simulink model "Buck_Control_Sim"  (R2023b)
settings: Solver=ode23t  StartTime=0.0  StopTime=20e-3  RelTol=1e-6
undefined symbols (not defined in the file): C, C1_dl_Den, C1_dl_Num, C1_sl_Den, C1_sl_Num, C2_dl_Den, C2_dl_Num, C2_dlh_Den, C2_dlh_Num, fs, L, R, Vg
libraries: spsSeriesRLCBranchLib x9, spsCurrentMeasurementLib x3, spsDiodeLib x3, spsIdealSwitchLib x3, spsMeanLib x3, eePwmGenerator x3, spsDCVoltageSourceLib x3, spsVoltageMeasurementLib x3, slpidlib x1, sps_lib x1
settings Model: Creator=Lucas  LastModifiedBy=Lucas
settings SolverCC: ZeroCrossAlgorithm=Adaptive
settings DebuggingCC: IgnoredZcDiagnostic=none

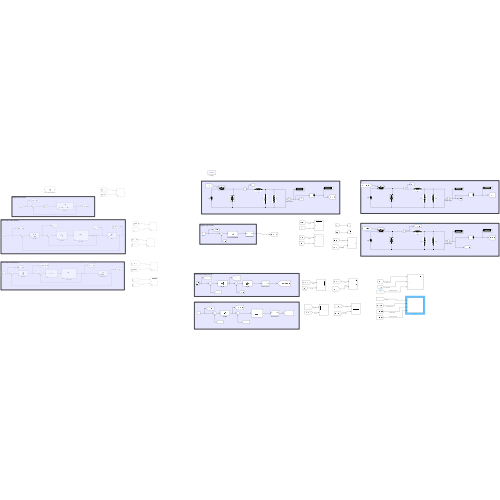
[thumbnail: Simulink's stored preview of the top-level diagram]
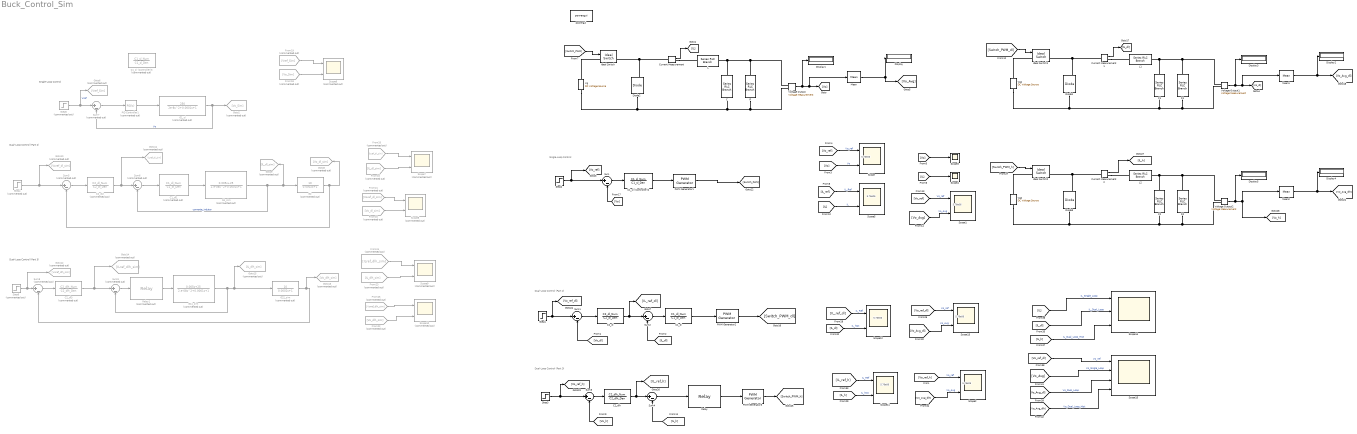
== system Buck_Control_Sim ==
  note: 5.76e06
  note: Single-Loop Control
  note: Dual-Loop Control (Part 2)
  note: 5.76e06
  note: Dual-Loop Control (Part 3)
  note: 5.76e06
  note: Dual-Loop Control (Part 2)
  note: Single-Loop Control
  note: Dual-Loop Control (Part 3)
  note: 5.76e06
  note: 5.76e06
  note: 5.76e06
  note: 5.76e06
  C : spsSeriesRLCBranchLib/Series RLC Branch  LConnTagsString=__new0  RConnTagsString=__new0  BranchType=C  Resistance=1  Inductance=L  SetiL0=off  InitialCurrent=0  Capacitance=C  Setx0=off  InitialVoltage=0  Measurements=None
  C1 : spsSeriesRLCBranchLib/Series RLC Branch  LConnTagsString=__new0  RConnTagsString=__new0  BranchType=C  Resistance=1  Inductance=L  SetiL0=off  InitialCurrent=0  Capacitance=C  Setx0=off  InitialVoltage=0  Measurements=None
  C1_dl : TransferFcn  Numerator=C1_dl_Num  Denominator=C1_dl_Den
  C1_dl1 : TransferFcn  Commented=on  Numerator=C1_dl_Num  Denominator=C1_dl_Den
  C1_sl (Controller)2 : TransferFcn  Numerator=C1_sl_Num  Denominator=C1_sl_Den
  C1_sl (Controller)3 : TransferFcn  Commented=on  Numerator=C1_sl_Num  Denominator=C1_sl_Den
  C2 : spsSeriesRLCBranchLib/Series RLC Branch  LConnTagsString=__new0  RConnTagsString=__new0  BranchType=C  Resistance=1  Inductance=L  SetiL0=off  InitialCurrent=0  Capacitance=C  Setx0=off  InitialVoltage=0  Measurements=None
  C2_dl : TransferFcn  Numerator=C2_dl_Num  Denominator=C2_dl_Den
  C2_dl2 : TransferFcn  Commented=on  Numerator=C2_dl_Num  Denominator=C2_dl_Den
  C2_dl3 : TransferFcn  Commented=on  Numerator=C2_dlh_Num  Denominator=C2_dlh_Den
  C2_dlh : TransferFcn  Numerator=C2_dlh_Num  Denominator=C2_dlh_Den
  Current Measurement : spsCurrentMeasurementLib/Current Measurement  PhasorSimulation=off  OutputType=Complex  PSBequivalent=0
  Current Measurement1 : spsCurrentMeasurementLib/Current Measurement  PhasorSimulation=off  OutputType=Complex  PSBequivalent=0
  Current Measurement2 : spsCurrentMeasurementLib/Current Measurement  PhasorSimulation=off  OutputType=Complex  PSBequivalent=0
  Diode1 : spsDiodeLib/Diode  Ron=0.00001  Lon=0  Vf=0  IC=0  UseSnubber=0  Rs=inf  Cs=inf  Measurements=on
  Diode2 : spsDiodeLib/Diode  Ron=0.00001  Lon=0  Vf=0  IC=0  UseSnubber=0  Rs=inf  Cs=inf  Measurements=on
  Diode3 : spsDiodeLib/Diode  Ron=0.00001  Lon=0  Vf=0  IC=0  UseSnubber=0  Rs=inf  Cs=inf  Measurements=on
  Display{,1..5} (6 alike) : Display
  From15 : From  Commented=on  GotoTag=Vo_dl_sim
  From16 : From  Commented=on  GotoTag=IL_dl_sim
  From18 : From  Commented=on  GotoTag=Vo_Sim
  From19 : From  Commented=on  GotoTag=Vref_Sim
  From20 : From  Commented=on  GotoTag=ILref_dl_sim
  From21 : From  Commented=on  GotoTag=Voref_dl_sim
  From22 : From  Commented=on  GotoTag=Vo_dlh_sim
  From23 : From  Commented=on  GotoTag=IL_dlh_sim
  From24 : From  Commented=on  GotoTag=ILref_dlh_sim
  From25 : From  Commented=on  GotoTag=Voref_dlh_sim
  G11_sim : TransferFcn  Commented=on  Numerator=[0 0.005 25]  Denominator=[2.e-08 0.0001 1]
  G1_sim : TransferFcn  Commented=on  Numerator=[0 0.005 25]  Denominator=[2.e-08 0.0001 1]
  G1_sl : TransferFcn  Commented=on  Numerator=[250]  Denominator=[2e-8 0.0001 1]
  G2 : TransferFcn  Commented=on  Numerator=[0,10]  Denominator=[0.0002 1]
  G22_sim : TransferFcn  Commented=on  Numerator=[0,10]  Denominator=[0.0002 1]
  Goto10 : Goto  Commented=on  GotoTag=Voref_dl_sim
  Goto11 : Goto  Commented=on  GotoTag=ILref_dl_sim
  Goto12 : Goto  Commented=on  GotoTag=Voref_dlh_sim
  Goto13 : Goto  Commented=on  GotoTag=Vo_dlh_sim
  Goto14 : Goto  Commented=on  GotoTag=ILref_dlh_sim
  Goto15 : Goto  Commented=on  GotoTag=IL_dlh_sim
  Goto2 : Goto  Commented=on  GotoTag=Vo_Sim
  Goto6 : Goto  Commented=on  GotoTag=Vref_Sim
  Goto8 : Goto  Commented=on  GotoTag=Vo_dl_sim
  Goto9 : Goto  Commented=on  GotoTag=IL_dl_sim
  Ideal Switch : spsIdealSwitchLib/Ideal Switch  Ron=0.001  Lon=0  IC=0  Rs=1e5  Cs=inf  Measurements=on
  Ideal Switch1 : spsIdealSwitchLib/Ideal Switch  Ron=0.001  Lon=0  IC=0  Rs=1e5  Cs=inf  Measurements=on
  Ideal Switch2 : spsIdealSwitchLib/Ideal Switch  Ron=0.001  Lon=0  IC=0  Rs=1e5  Cs=inf  Measurements=on
  L : spsSeriesRLCBranchLib/Series RLC Branch  LConnTagsString=__new0  RConnTagsString=__new0  BranchType=L  Resistance=1  Inductance=L  SetiL0=off  InitialCurrent=0  Capacitance=1e-6  Setx0=off  InitialVoltage=0  Measurements=None
  L1 : spsSeriesRLCBranchLib/Series RLC Branch  LConnTagsString=__new0  RConnTagsString=__new0  BranchType=L  Resistance=1  Inductance=L  SetiL0=off  InitialCurrent=0  Capacitance=1e-6  Setx0=off  InitialVoltage=0  Measurements=None
  L2 : spsSeriesRLCBranchLib/Series RLC Branch  LConnTagsString=__new0  RConnTagsString=__new0  BranchType=L  Resistance=1  Inductance=L  SetiL0=off  InitialCurrent=0  Capacitance=1e-6  Setx0=off  InitialVoltage=0  Measurements=None
  Mean : spsMeanLib/Mean  Freq=fs  Vinit=0  Ts=0
  Mean1 : spsMeanLib/Mean  Freq=fs  Vinit=0  Ts=0
  Mean2 : spsMeanLib/Mean  Freq=fs  Vinit=0  Ts=0
  PID Controller1 : slpidlib/PID Controller  Commented=on  Controller=PID  Form=Parallel  TimeDomain=Continuous-time  UseExternalTs=off  SampleTime=-1  IntegratorMethod=Forward Euler  FilterMethod=Forward Euler  ControllerParametersSource=internal  P=0  I=6.07  UseKiTs=off  D=0  N=100  UseFilter=on  TunerSelectOption=Transfer Function Based (PID Tuner App)  InitialConditionSource=internal  InitialConditionForIntegrator=0  InitialConditionForFilter=0  DifferentiatorICPrevScaledInput=0  ExternalReset=none  TrackingMode=off  Kt=1  LimitOutput=off  SatLimitsSource=internal  UpperSaturationLimit=inf  LowerSaturationLimit=-inf  LinearizeAsGain=on  AntiWindupMode=none  Kb=1  LimitIntegrator=off  UpperIntegratorSaturationLimit=inf  LowerIntegratorSaturationLimit=-inf  POutMin=[]  POutMax=[]  IOutMin=[]  IOutMax=[]  DOutMin=[]  DOutMax=[]  NOutMin=[]  NOutMax=[]  SumOutMin=[]  SumOutMax=[]  SaturationOutMin=[]  SaturationOutMax=[]  PParamMin=[]  PParamMax=[]  IParamMin=[]  IParamMax=[]  DParamMin=[]  DParamMax=[]  NParamMin=[]  NParamMax=[]  KbParamMin=[]  KbParamMax=[]  KtParamMin=[]  KtParamMax=[]  KbOutMin=[]  KbOutMax=[]  KtOutMin=[]  KtOutMax=[]  IntegratorOutMin=[]  IntegratorOutMax=[]  FilterOutMin=[]  FilterOutMax=[]  SumI1OutMin=[]  SumI1OutMax=[]  SumI2OutMin=[]  SumI2OutMax=[]  SumI3OutMin=[]  SumI3OutMax=[]  SumI4OutMin=[]  SumI4OutMax=[]  SumDOutMin=[]  SumDOutMax=[]  DifferentiatorOutMin=[]  DifferentiatorOutMax=[]  FilterDiffOutCoefMin=[]  FilterDiffOutCoefMax=[]  ReciprocalOutMin=[]  ReciprocalOutMax=[]  SumDenOutMin=[]  SumDenOutMax=[]  SumNumOutMin=[]  SumNumOutMax=[]  DivideOutMin=[]  DivideOutMax=[]  UdiffTsProdOutMin=[]  UdiffTsProdOutMax=[]  NTsProdOutMin=[]  NTsProdOutMax=[]  UintegralTsProdOutMin=[]  UintegralTsProdOutMax=[]  UngainTsProdOutMin=[]  UngainTsProdOutMax=[]  ClampingZeroOutDataTypeStr=Inherit: Inherit via back propagation  ClampingZeroOutMin=[]  ClampingZeroOutMax=[]  FilterDenConstantOutDataTypeStr=Inherit: Inherit via back propagation  FilterDenConstantOutMin=[]  FilterDenConstantOutMax=[]  PCopyOutDataTypeStr=Inherit: Inherit via back propagation  PCopyOutMin=[]  PCopyOutMax=[]  NCopyOutDataTypeStr=Inherit: Inherit via back propagation  NCopyOutMin=[]  NCopyOutMax=[]  IntegratorContinuousStateAttributes=''  IntegratorStateMustResolveToSignalObject=off  IntegratorRTWStateStorageClass=Auto  FilterContinuousStateAttributes=''  FilterStateMustResolveToSignalObject=off  FilterRTWStateStorageClass=Auto  ParallelPVariant=InternalParameters  IdealPVariant=Disabled  IVariant=InternalParameters  DVariant=InternalParameters  IntegratorVariant=Continuous  SatVariant=Disabled  AWVariant=Passthrough  PCopyVariant=Disabled  TRVariant=Disabled  FdbkBlocksVariant=Forward  IdealPFdbkVariant=Disabled  SatFdbkVariant=Disabled  DerivativeFilterVariant=ContFilter  NVariant=InternalParameters  NCopyVariant=Disabled  FilterICVariant=InternalICsFilter  IntegratorICVariant=InternalICs  ExternalResetVariant=Disabled  TRSumVariant=Passthrough  SumFdbkVariant=Disabled  SumVariant=Sum_PID  TsampFilterVariant=InternalTs  TsampNgainVariant=Passthrough  TsampIntegralVariant=Disabled_SignalSpec  ExternalSaturationOutDataTypeStr=Inherit: Same as second input
  PWM Generator1 : eePwmGenerator/PWM Generator  CarrCount=Up  Tper=1/fs  Tdelay=0  Ts=0
  PWM Generator2 : eePwmGenerator/PWM Generator  CarrCount=Up  Tper=1/fs  Tdelay=0  Ts=0
  PWM Generator3 : eePwmGenerator/PWM Generator  CarrCount=Up  Tper=1/fs  Tdelay=0  Ts=0
  R : spsSeriesRLCBranchLib/Series RLC Branch  LConnTagsString=__new0  RConnTagsString=__new0  BranchType=R  Resistance=R  Inductance=L  SetiL0=off  InitialCurrent=0  Capacitance=1e-6  Setx0=off  InitialVoltage=0  Measurements=None
  R1 : spsSeriesRLCBranchLib/Series RLC Branch  LConnTagsString=__new0  RConnTagsString=__new0  BranchType=R  Resistance=R  Inductance=L  SetiL0=off  InitialCurrent=0  Capacitance=1e-6  Setx0=off  InitialVoltage=0  Measurements=None
  R2 : spsSeriesRLCBranchLib/Series RLC Branch  LConnTagsString=__new0  RConnTagsString=__new0  BranchType=R  Resistance=R  Inductance=L  SetiL0=off  InitialCurrent=0  Capacitance=1e-6  Setx0=off  InitialVoltage=0  Measurements=None
  Relay : Relay  OnSwitchValue=0.1  OffSwitchValue=0  OnOutputValue=200
  Relay1 : Relay  Commented=on  OnSwitchValue=0.1  OffSwitchValue=0  OnOutputValue=200
  Scope{,1..2,5,11..13} (7 alike) : Scope  NumInputPorts=2
  Scope{6..10} (5 alike) : Scope  Commented=on  NumInputPorts=2
  Scope14 : Scope  NumInputPorts=3
  Scope15 : Scope  NumInputPorts=4
  Scope3 : Scope
  Scope4 : Scope
  Step1 : Step  Time=10e-3  Before=60  After=66  SampleTime=0
  Step2 : Step  Time=10e-3  Before=60  After=66  SampleTime=0
  Step3 : Step  Time=10e-3  Before=60  After=66  SampleTime=0
  Step4 : Step  Commented=on  Time=6e-3  Before=60  After=66  SampleTime=0
  Step5 : Step  Commented=on  Time=6e-3  Before=60  After=66  SampleTime=0
  Step6 : Step  Commented=on  Time=6e-3  Before=60  After=66  SampleTime=0
  Sum{,1..4} (5 alike) : Sum  Inputs=|+-
  Sum{5..9} (5 alike) : Sum  Commented=on  Inputs=|+-
  Vg : spsDCVoltageSourceLib/DC Voltage Source  Amplitude=Vg  Measurements=None
  Vg1 : spsDCVoltageSourceLib/DC Voltage Source  Amplitude=Vg  Measurements=None
  Vg2 : spsDCVoltageSourceLib/DC Voltage Source  Amplitude=Vg  Measurements=None
  Voltage Output : spsVoltageMeasurementLib/Voltage Measurement  PhasorSimulation=off  OutputType=Complex  PSBequivalent=0
  Voltage Output1 : spsVoltageMeasurementLib/Voltage Measurement  PhasorSimulation=off  OutputType=Complex  PSBequivalent=0
  Voltage Output2 : spsVoltageMeasurementLib/Voltage Measurement  PhasorSimulation=off  OutputType=Complex  PSBequivalent=0
  powergui : sps_lib/powergui  Priority=1  SimulationMode=Continuous  SampleTime=50e-6  frequency=60  Iterations=50  frequencyindice=0  Pbase=100e6  ErrMax=1e-4  UnitsV=kV  UnitsW=MW  buscounter=0  FunctionMessages=off  echomessages=off  EnableUseOfTLC=off  CurrentSourceSwitches=off  DisableSnubberDevices=off  DisableRonSwitches=off  DisableVfSwitches=off  DisplayEquations=off  AutomaticDiscreteSolvers=off  SolverType=Tustin/Backward Euler (TBE)  Interpol=off  ExternalGateDelay=off  methode=off  Ts=100  x0status=blocks  SPID=on  SwTol=0  HookPort=off  NonlinearTolerance=1e-4  nMaxIteration=100  ContinueOnMaxIteration=off  RestoreLinks=warning  ResistiveCurrentMeasurement=off  Frange=[0:2:500]  Ylog=off  Xlog=on  ShowGrid=off  save=off  variable=ZData  structure=0  ZoomFFT=off  StartTime=0.0  cycles=1  DisplayStyle=1  fundamental=60  FreqAxis=off  MaxFrequency=1000  frequencyindicesteady=1  RmsSteady=1  display=off
  wires:
  Step2/1 -> [Vo_ref], Sum/1
  Voltage Output/1 -> Display1/1, Mean/1, [Vo]
  Step1/1 -> Sum1/1, [Vo_ref_dl]
  Current Measurement/1 -> [IL]
  [Vo] -> Scope/2  "Vo"
  [Vo_ref] -> Scope/1  "Vo_ref"
  Sum1/1 -> C2_dl/1
  [Vo_dl] -> Sum1/2
  [IL_dl] -> Sum2/2
  C2_dl/1 -> [IL_ref_dl], Sum2/1
  Sum2/1 -> C1_dl/1
  [Vo] -> Scope3/1
  [IL] -> Scope4/1
  Sum/1 -> C1_sl (Controller)2/1
  [IL_ref] -> Scope5/1  "IL_Ref"
  [IL] -> Scope5/2  "IL"
  [IL_h] -> Sum4/2
  [Vo_h] -> Sum3/2
  Sum4/1 -> Relay/1
  Step3/1 -> [Vo_ref_h], Sum3/1
  C1_dl/1 -> PWM Generator2/1
  Mean/1 -> Display/1, [Vo_Avg]
  [Vo_ref] -> Scope1/1  "Vo_ref"
  [Vo_Avg] -> Scope1/2  "Vo_Avg"
  C1_sl (Controller)2/1 -> PWM Generator1/1
  Relay/1 -> PWM Generator3/1
  C2_dlh/1 -> Sum4/1, [IL_ref_h]
  Sum3/1 -> C2_dlh/1
  C2_dl2/1 -> Goto11/1, Sum6/1
  Sum6/1 -> C1_dl1/1
  Step4/1 -> Goto10/1, Sum5/1
  Sum5/1 -> C2_dl2/1
  C1_dl1/1 -> G1_sim/1
  G1_sim/1 -> Goto9/1, G2/1, Sum6/2  "corrente_indutor"
  [Vo] -> Sum/2
  G1_sl/1 -> Sum7/2, Goto2/1  "Vo"
  Step5/1 -> Goto6/1, Sum7/1  "Vref"
  PID Controller1/1 -> G1_sl/1
  Sum7/1 -> PID Controller1/1
  From19/1 -> Scope6/1
  From18/1 -> Scope6/2
  G2/1 -> Sum5/2, Goto8/1
  From21/1 -> Scope8/1
  From15/1 -> Scope8/2
  From20/1 -> Scope7/1
  From16/1 -> Scope7/2
  C2_dl3/1 -> Goto14/1, Sum9/1
  Sum9/1 -> Relay1/1
  G11_sim/1 -> Goto15/1, G22_sim/1, Sum9/2
  Relay1/1 -> G11_sim/1
  Step6/1 -> Goto12/1, Sum8/1
  Sum8/1 -> C2_dl3/1
  G22_sim/1 -> Goto13/1, Sum8/2
  From23/1 -> Scope9/2
  From22/1 -> Scope10/2
  From25/1 -> Scope10/1
  From24/1 -> Scope9/1
  [Switch_PWM] -> Ideal Switch/1
  PWM Generator2/1 -> [Switch_PWM_dl]
  [Switch_PWM_dl] -> Ideal Switch1/1
  Current Measurement1/1 -> [IL_dl]
  Voltage Output1/1 -> Display3/1, Mean1/1, [Vo_dl]
  Mean1/1 -> Display2/1, [Vo_Avg_dl]
  [Switch_PWM_h] -> Ideal Switch2/1
  Current Measurement2/1 -> [IL_h]
  Voltage Output2/1 -> Display5/1, [Vo_h], Mean2/1
  Mean2/1 -> Display4/1, [Vo_Avg_dlh]
  PWM Generator1/1 -> [Switch_PWM]
  PWM Generator3/1 -> [Switch_PWM_h]
  [Vo_Avg_dlh] -> Scope2/2  "Vo_Avg"
  [Vo_ref_h] -> Scope2/1  "Vo_ref"
  [IL_ref_h] -> Scope11/1  "IL_Ref"
  [IL_h] -> Scope11/2  "IL_hist"
  [Vo_Avg_dl] -> Scope13/2  "Vo_Avg"
  [Vo_ref_dl] -> Scope13/1  "Vo_ref"
  [IL_dl] -> Scope12/2  "IL_hist"
  [IL_ref_dl] -> Scope12/1  "IL_Ref"
  [IL_dl] -> Scope14/2  "IL_Dual_Loop"
  [IL_h] -> Scope14/3  "IL_Dual_Loop_Hist"
  [IL] -> Scope14/1  "IL_Single_Loop"
  [Vo_Avg_dlh] -> Scope15/4  "Vo_Dual_Loop_Hist"
  [Vo_Avg_dl] -> Scope15/3  "Vo_Dual_Loop"
  [Vo_ref_dl] -> Scope15/1  "Vo_ref"
  [Vo_Avg] -> Scope15/2  "Vo_Single_Loop"
  connections:
  R/LConn1 -- Voltage Output/LConn1 -- C/LConn1 -- L/RConn1
  R/RConn1 -- Voltage Output/LConn2 -- Vg/LConn1 -- Diode2/LConn1 -- C/RConn1
  Current Measurement/LConn1 -- Diode2/RConn1 -- Ideal Switch/RConn1
  Ideal Switch/LConn1 -- Vg/RConn1
  Current Measurement/RConn1 -- L/LConn1
  L1/RConn1 -- C1/LConn1 -- R1/LConn1 -- Voltage Output1/LConn1
  Ideal Switch1/RConn1 -- Current Measurement1/LConn1 -- Diode1/RConn1
  C1/RConn1 -- Vg1/LConn1 -- Diode1/LConn1 -- R1/RConn1 -- Voltage Output1/LConn2
  Current Measurement1/RConn1 -- L1/LConn1
  Ideal Switch1/LConn1 -- Vg1/RConn1
  L2/RConn1 -- C2/LConn1 -- R2/LConn1 -- Voltage Output2/LConn1
  Ideal Switch2/RConn1 -- Current Measurement2/LConn1 -- Diode3/RConn1
  C2/RConn1 -- Vg2/LConn1 -- Diode3/LConn1 -- R2/RConn1 -- Voltage Output2/LConn2
  Current Measurement2/RConn1 -- L2/LConn1
  Ideal Switch2/LConn1 -- Vg2/RConn1
